simulink model "RL_TTS1_TOP_SIM_6E8X0"  (R2021b)
settings: Solver=VariableStepAuto  StartTime=0.0  StopTime=800  RelTol=1e-3
settings Model: Creator=whendrix  LastModifiedBy=20191255
settings SolverCC: AlgebraicLoopSolver=TrustRegion
settings DebuggingCC: SFMachineParentedDataDiag=warning
settings SFSimCC: CustomCodeUndefinedFunction=UseInterfaceOnly

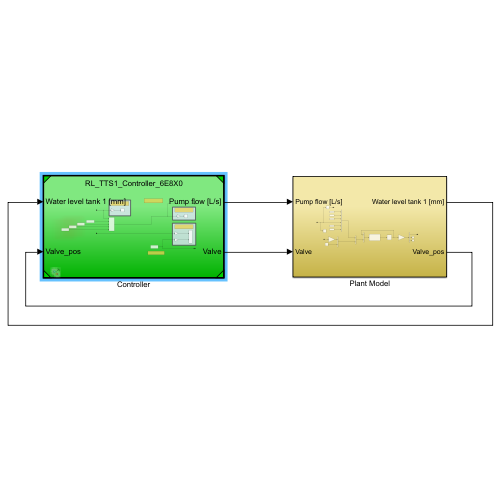
[thumbnail: Simulink's stored preview of the top-level diagram]
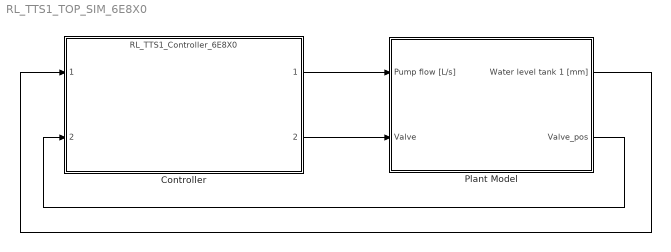
== system RL_TTS1_TOP_SIM_6E8X0 ==
  Controller : ModelReference  ModelNameDialog=RL_TTS1_Controller_6E8X0.slx  SimulationMode=Normal  ModelReferenceVersion=5.9
  Plant Model : Subsystem
  wires:
  Plant Model/1(Water level tank 1 [mm]) -> Controller/1
  Controller/1 -> Plant Model/1(Pump flow [L/s])
  Controller/2 -> Plant Model/2(Valve)
  Plant Model/2(Valve_pos) -> Controller/2

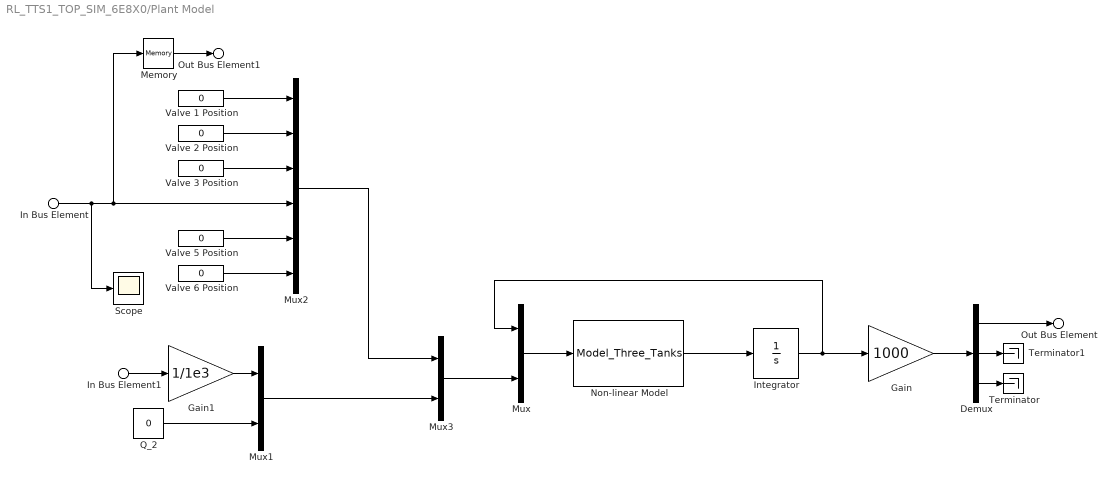
== system RL_TTS1_TOP_SIM_6E8X0/Plant Model ==
  In Bus Element1 : Inport  PortName=Pump flow [L/s]  Element=Left
  In Bus Element : Inport  Port=2  PortName=Valve  Element=LD_posref
  Demux : Demux  Outputs=3
  Gain : Gain  Gain=1000
  Gain1 : Gain  Gain=1/1e3
  Integrator : Integrator  InitialCondition=[ 0 0 0]  LimitOutput=on  LowerSaturationLimit=[0 0 0]  ZeroCross=off
  Memory : Memory
  Mux : Mux  Inputs=2
  Mux1 : Mux  Inputs=2
  Mux2 : Mux  Inputs=6
  Mux3 : Mux  Inputs=2
  "Non-linear Model " : MATLABFcn  MATLABFcn=Model_Three_Tanks  OutputSignalType=real
  Q_2 : Constant  Value=0
  Scope : Scope
  Terminator : Terminator
  Terminator1 : Terminator
  Valve 1 Position : Constant  Value=0
  Valve 2 Position : Constant  Value=0
  Valve 3 Position : Constant  Value=0
  Valve 5 Position : Constant  Value=0
  Valve 6 Position : Constant  Value=0
  Out Bus Element : Outport  PortName=Water level tank 1 [mm]  Element=Left
  Out Bus Element1 : Outport  Port=2  PortName=Valve_pos  Element=LD_pos
  wires:
  Mux2/1 -> Mux3/1
  Integrator/1 -> Mux/1, Gain/1
  Mux1/1 -> Mux3/2
  Mux/1 -> "Non-linear Model "/1
  "Non-linear Model "/1 -> Integrator/1
  Q_2/1 -> Mux1/2
  Mux3/1 -> Mux/2
  In Bus Element1/1 -> Gain1/1
  In Bus Element/1 -> Scope/1, Memory/1, Mux2/4
  Valve 1 Position/1 -> Mux2/1
  Valve 2 Position/1 -> Mux2/2
  Valve 3 Position/1 -> Mux2/3
  Valve 5 Position/1 -> Mux2/5
  Valve 6 Position/1 -> Mux2/6
  Gain/1 -> Demux/1
  Demux/3 -> Terminator/1
  Demux/2 -> Terminator1/1
  Gain1/1 -> Mux1/1
  Demux/1 -> Out Bus Element/1
  Memory/1 -> Out Bus Element1/1
